simulink model "Quad_sim"  (Simulink 10.1)
settings: Solver=FixedStepAuto  StartTime=0.0  StopTime=10  FixedStep=0.01  RelTol=1e-3
values from neighbouring files (symbols this model uses):
  g = 9.81    [fcn1.m]
undefined symbols (not defined in the file or in its folder): Jr, Jx, Jy, Jz, Kd, Kd_p, Kd_q, Kd_r, Kdx, Kdy, Kdz, Ki_p, Ki_q, Ki_r, Kp_p, Kp_q, Kp_r, KT, l, m, max_motor_speed, min_motor_speed, p_max, phi_max, q_max, r_max, theta_max, U1_max, U1_min, U2_max, U2_min, U3_max, U3_min, U4_max, U4_min
settings Model: Creator=Jarvis  LastModifiedBy=nikhil
settings DataIOCC: SaveFormat=Dataset
settings OptimizationCC: LifeSpan=auto
settings DebuggingCC: UnderspecifiedInitializationDetection=Simplified  MergeDetectMultiDrivingBlocksExec=error  SFUnexpectedBacktrackingDiag=error  SFNoUnconditionalDefaultTransitionDiag=error  SFExecutionAtInitializationDiag=warning
settings HardwareCC: ProdBitPerPointer=64  ProdBitPerSizeT=64  ProdBitPerPtrDiffT=64  ProdLargestAtomicFloat=Float  ProdIntDivRoundTo=Zero  ProdEndianess=LittleEndian  ProdWordSize=64  ProdHWDeviceType=Intel->x86-64 (Windows64)
settings ModelReferenceCC: PropagateSignalLabelsOutOfModel=on
settings GRTTargetCC: TargetLangStandard=C99 (ISO)  CombineOutputUpdateFcns=on  GRTInterface=off
settings ConfigComp: CovMetricSettings=dwe  CovHtmlReporting=off  CovSaveCumulativeToWorkspaceVar=off  CovSaveSingleToWorkspaceVar=off  CovExternalEMLEnable=on

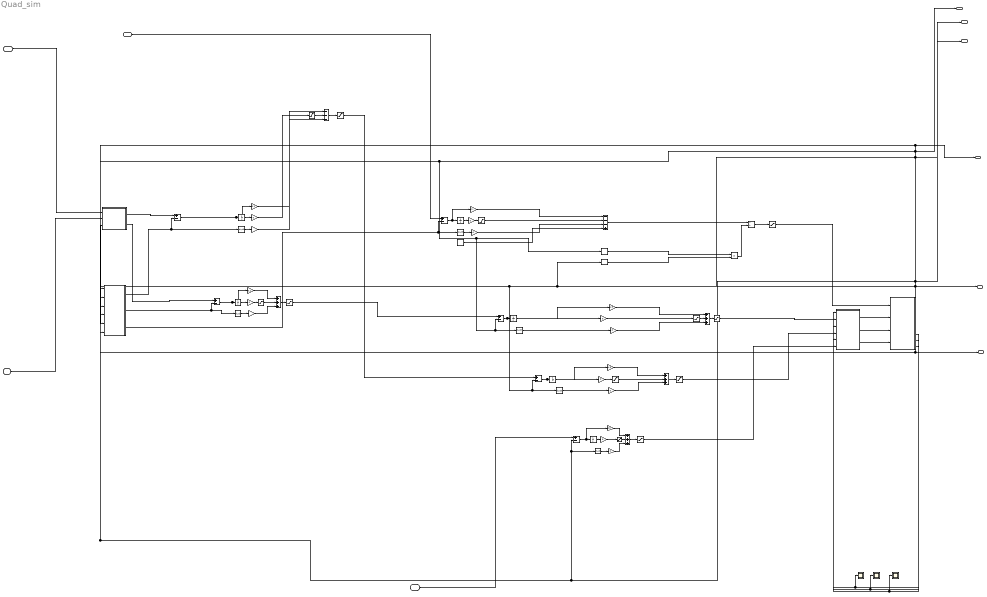
== system Quad_sim ==
  note: Psi PID
  note: Theta PID
  note: Phi PID
  note: Z PID
  note: Attitude/Altitude
      | PID Controller
  note: y control
  note: x control
  note: Position Control
  Xd : Inport
  Yd : Inport  Port=2
  Zd : Inport  Port=3
  Psid : Inport  Port=4
  Angular Rate  PID Controller : Subsystem
  "Current Positions from GF -> BF" : Subsystem
  Derivative{,1..5} (6 alike) : Derivative
  "Desired Positions from GF -> BF" : Subsystem
  Divide : Product  Inputs=*/
  Integrator{,1..5} (6 alike) : Integrator
  Kd : Gain  Gain=-0.1
  Kd1 : Gain  Gain=-0.1
  Kd2 : Gain  Gain=-4
  Kd3 : Gain  Gain=0
  Kd4 : Gain  Gain=0
  Kd5 : Gain  Gain=0
  Ki{,1..5} (6 alike) : Gain  Gain=0
  Kp : Gain  Gain=0.1
  Kp1 : Gain  Gain=0.1
  Kp2 : Gain  Gain=1.5625
  Kp3 : Gain  Gain=4.5
  Kp4 : Gain  Gain=4.5
  Kp5 : Gain  Gain=10
  Product : Product  RndMeth=Zero
  Psi Error : Sum  Inputs=+-
  Psi Error1 : Sum  Inputs=+-
  Quadrotor System : Subsystem
  Saturation : Saturate  UpperLimit=U1_max  LowerLimit=U1_min  ZeroCross=off
  Saturation1 : Saturate  UpperLimit=theta_max  LowerLimit=-theta_max  ZeroCross=off
  Saturation10 : Saturate  UpperLimit=r_max  LowerLimit=-r_max  ZeroCross=off
  Saturation11 : Saturate  UpperLimit=r_max  LowerLimit=-r_max  ZeroCross=off
  Saturation2 : Saturate  UpperLimit=theta_max  LowerLimit=-theta_max  ZeroCross=off
  Saturation3 : Saturate  UpperLimit=phi_max  LowerLimit=-phi_max  ZeroCross=off
  Saturation4 : Saturate  UpperLimit=phi_max  LowerLimit=-phi_max  ZeroCross=off
  Saturation5 : Saturate  UpperLimit=U1_max  LowerLimit=U1_min  ZeroCross=off
  Saturation6 : Saturate  UpperLimit=p_max  LowerLimit=-p_max  ZeroCross=off
  Saturation7 : Saturate  UpperLimit=p_max  LowerLimit=-p_max  ZeroCross=off
  Saturation8 : Saturate  UpperLimit=q_max  LowerLimit=-q_max  ZeroCross=off
  Saturation9 : Saturate  UpperLimit=q_max  LowerLimit=-q_max  ZeroCross=off
  Sum : Sum  Inputs=---
  Sum{1,3..5} (4 alike) : Sum  Inputs=+++
  Sum2 : Sum  Inputs=---+
  Theta Error : Sum  Inputs=+-
  X Error : Sum  Inputs=+-
  Y Error : Sum  Inputs=+-
  cos Phi : Trigonometry  Operator=cos
  cos Theta : Trigonometry  Operator=cos
  ez : Sum  Inputs=+-
  mg : Constant  Value=m*g
  p_Out : Scope
  q_Out : Scope
  r_Out : Scope
  X : Outport
  Y : Outport  Port=2
  Z : Outport  Port=3
  Phi : Outport  Port=4
  Theta : Outport  Port=5
  Psi : Outport  Port=6
  wires:
  Quadrotor System/1(Z) -> Z/1, "Current Positions from GF -> BF"/3(Z)  "Z"
  Quadrotor System/2(Phi) -> Phi/1, "Current Positions from GF -> BF"/4(phi), Psi Error/2, Derivative3/1, cos Phi/1  "Phi"
  Quadrotor System/3(Theta) -> Theta/1, "Current Positions from GF -> BF"/5(theta), Theta Error/2, Derivative4/1, cos Theta/1  "Theta"
  Quadrotor System/4(Psi) -> Psi/1, "Desired Positions from GF -> BF"/3(psi), "Current Positions from GF -> BF"/6(Psi), Psi Error1/2, Derivative5/1  "Psi"
  Quadrotor System/5(X) -> X/1, "Current Positions from GF -> BF"/1(X)  "X"
  Quadrotor System/6(Y) -> Y/1, "Current Positions from GF -> BF"/2(Y)  "Y"
  Quadrotor System/7(p) -> Angular Rate  PID Controller/1(p), p_Out/1
  Quadrotor System/8(q) -> q_Out/1, Angular Rate  PID Controller/3(q)
  Quadrotor System/9(r) -> r_Out/1, Angular Rate  PID Controller/5(r)
  Angular Rate  PID Controller/1(U2) -> Quadrotor System/2(U2)
  Angular Rate  PID Controller/2(U3) -> Quadrotor System/3(U3)
  Angular Rate  PID Controller/3(U4) -> Quadrotor System/4(U4)
  Saturation7/1 -> Angular Rate  PID Controller/2(p desired)
  Saturation9/1 -> Angular Rate  PID Controller/4(q desired)
  Saturation11/1 -> Angular Rate  PID Controller/6(r desired)
  Psid/1 -> Psi Error1/1  "Psid"
  Zd/1 -> ez/1  "Zd"
  Xd/1 -> "Desired Positions from GF -> BF"/1(X_des)  "Xd"
  Yd/1 -> "Desired Positions from GF -> BF"/2(Y_des)  "Yd"
  Saturation/1 -> Quadrotor System/1(U1)
  Sum/1 -> Saturation2/1
  Derivative/1 -> Kd/1
  Kp/1 -> Sum/1  "x_kp"
  "Desired Positions from GF -> BF"/1(x_des) -> X Error/1
  X Error/1 -> Integrator/1, Kp/1
  Saturation1/1 -> Sum/2
  Ki/1 -> Saturation1/1  "x_ki"
  "Current Positions from GF -> BF"/1(x) -> X Error/2, Derivative/1
  Kd/1 -> Sum/3  "x_kd"
  Integrator/1 -> Ki/1
  Kp1/1 -> Sum1/1  "y_kp"
  Ki1/1 -> Saturation3/1  "y_ki"
  Derivative1/1 -> Kd1/1
  "Desired Positions from GF -> BF"/2(y_des) -> Y Error/1
  Saturation3/1 -> Sum1/2
  Sum1/1 -> Saturation4/1
  "Current Positions from GF -> BF"/2(y) -> Derivative1/1, Y Error/2
  Kd1/1 -> Sum1/3  "y_kd"
  Integrator1/1 -> Ki1/1
  Y Error/1 -> Integrator1/1, Kp1/1
  Saturation5/1 -> Sum2/2
  Ki2/1 -> Saturation5/1  "z_ki"
  Divide/1 -> Saturation/1
  Kd2/1 -> Sum2/3  "z_kd"
  mg/1 -> Sum2/4
  Sum2/1 -> Divide/1
  ez/1 -> Integrator2/1, Kp2/1
  Integrator2/1 -> Ki2/1
  Kp2/1 -> Sum2/1  "z_kp"
  Derivative2/1 -> Kd2/1
  "Current Positions from GF -> BF"/3(z) -> ez/2, Derivative2/1
  Product/1 -> Divide/2
  cos Theta/1 -> Product/2
  cos Phi/1 -> Product/1
  Sum3/1 -> Saturation7/1
  Saturation6/1 -> Sum3/2
  Ki3/1 -> Saturation6/1  "phi_ki"
  Kd3/1 -> Sum3/3  "phi_kd"
  Integrator3/1 -> Ki3/1
  Psi Error/1 -> Integrator3/1, Kp3/1
  Kp3/1 -> Sum3/1  "phi_kp"
  Derivative3/1 -> Kd3/1
  Saturation4/1 -> Psi Error/1
  Sum4/1 -> Saturation9/1
  Saturation8/1 -> Sum4/2
  Ki4/1 -> Saturation8/1  "theta_ki"
  Kd4/1 -> Sum4/3  "theta_kd"
  Integrator4/1 -> Ki4/1
  Theta Error/1 -> Integrator4/1, Kp4/1
  Kp4/1 -> Sum4/1  "theta_kp"
  Derivative4/1 -> Kd4/1
  Saturation2/1 -> Theta Error/1
  Sum5/1 -> Saturation11/1
  Saturation10/1 -> Sum5/2
  Ki5/1 -> Saturation10/1  "psi_ki"
  Kd5/1 -> Sum5/3  "psi_kd"
  Integrator5/1 -> Ki5/1
  Psi Error1/1 -> Integrator5/1, Kp5/1
  Kp5/1 -> Sum5/1  "psi_kp"
  Derivative5/1 -> Kd5/1

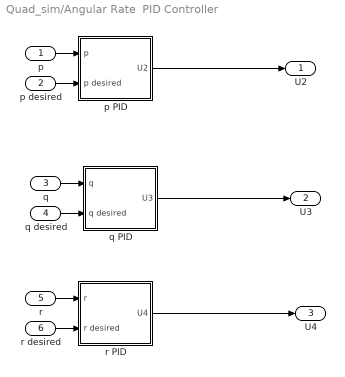
== system Quad_sim/Angular Rate  PID Controller ==
  p : Inport
  p desired : Inport  Port=2
  q : Inport  Port=3
  q desired : Inport  Port=4
  r : Inport  Port=5
  r desired : Inport  Port=6
  p PID : Subsystem
  q PID : Subsystem
  r PID : Subsystem
  U2 : Outport
  U3 : Outport  Port=2
  U4 : Outport  Port=3
  wires:
  p PID/1(U2) -> U2/1
  q PID/1(U3) -> U3/1
  r PID/1(U4) -> U4/1
  p/1 -> p PID/1(p)
  p desired/1 -> p PID/2(p desired)
  q/1 -> q PID/1(q)
  q desired/1 -> q PID/2(q desired)
  r/1 -> r PID/1(r)
  r desired/1 -> r PID/2(r desired)

== system Quad_sim/Current Positions from GF -> BF ==
  X : Inport
  Y : Inport  Port=2
  Z : Inport  Port=3
  phi : Inport  Port=4
  theta : Inport  Port=5
  Psi : Inport  Port=6
  x_bodyframe : Subsystem
  y_bodyframe : Subsystem
  z_bodyframe : Subsystem
  x : Outport
  y : Outport  Port=2
  z : Outport  Port=3
  wires:
  X/1 -> z_bodyframe/4(X), y_bodyframe/4(X), x_bodyframe/4(X)
  Y/1 -> z_bodyframe/5(Y), y_bodyframe/5(Y), x_bodyframe/5(Y)
  Z/1 -> z_bodyframe/6(Z), y_bodyframe/6(Z), x_bodyframe/6(Z)
  phi/1 -> z_bodyframe/1(phi), y_bodyframe/1(phi), x_bodyframe/1(phi)
  theta/1 -> z_bodyframe/2(theta), y_bodyframe/2(theta), x_bodyframe/2(theta)
  Psi/1 -> y_bodyframe/3(psi), x_bodyframe/3(psi), z_bodyframe/3(psi)
  x_bodyframe/1(x) -> x/1
  y_bodyframe/1(y) -> y/1
  z_bodyframe/1(z) -> z/1

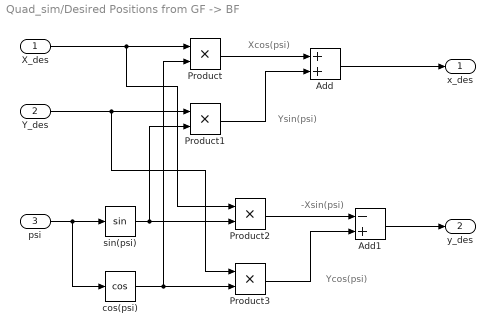
== system Quad_sim/Desired Positions from GF -> BF ==
  note: Xcos(psi)
  note: Ysin(psi)
  note: Ycos(psi)
  note: -Xsin(psi)
  X_des : Inport
  Y_des : Inport  Port=2
  psi : Inport  Port=3
  Add : Sum
  Add1 : Sum  Inputs=-+
  Product{,1..3} (4 alike) : Product
  cos(psi) : Trigonometry  Operator=cos
  sin(psi) : Trigonometry
  x_des : Outport
  y_des : Outport  Port=2
  wires:
  psi/1 -> cos(psi)/1, sin(psi)/1
  X_des/1 -> Product2/1, Product/1
  cos(psi)/1 -> Product3/2, Product/2
  Y_des/1 -> Product3/1, Product1/1
  Product/1 -> Add/1
  sin(psi)/1 -> Product2/2, Product1/2
  Product1/1 -> Add/2
  Add/1 -> x_des/1
  Product2/1 -> Add1/1
  Product3/1 -> Add1/2
  Add1/1 -> y_des/1

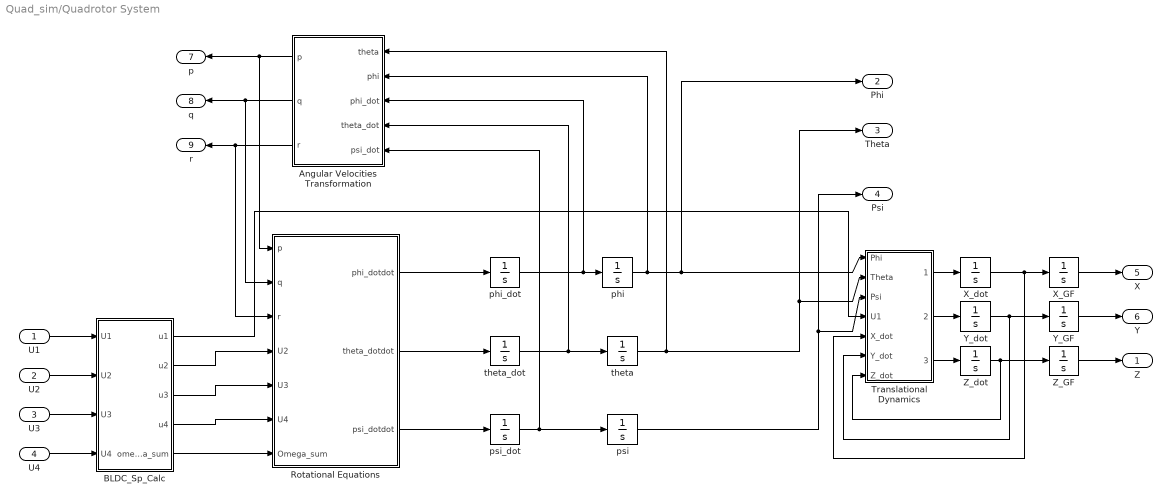
== system Quad_sim/Quadrotor System ==
  U1 : Inport
  U2 : Inport  Port=2
  U3 : Inport  Port=3
  U4 : Inport  Port=4
  Angular Velocities Transformation : Subsystem
  BLDC_Sp_Calc : Subsystem
  Rotational Equations : Subsystem
  Translational Dynamics : Subsystem
  X_GF : Integrator
  X_dot : Integrator
  Y_GF : Integrator
  Y_dot : Integrator
  Z_GF : Integrator
  Z_dot : Integrator
  phi : Integrator  ZeroCross=off
  phi_dot : Integrator
  psi : Integrator  ZeroCross=off
  psi_dot : Integrator  ZeroCross=off
  theta : Integrator  ZeroCross=off
  theta_dot : Integrator  ZeroCross=off
  Z : Outport
  Phi : Outport  Port=2
  Theta : Outport  Port=3
  Psi : Outport  Port=4
  X : Outport  Port=5
  Y : Outport  Port=6
  p : Outport  Port=7
  q : Outport  Port=8
  r : Outport  Port=9
  wires:
  U1/1 -> BLDC_Sp_Calc/1(U1)
  Angular Velocities Transformation/3(r) -> r/1, Rotational Equations/3(r)
  Angular Velocities Transformation/2(q) -> q/1, Rotational Equations/2(q)
  Angular Velocities Transformation/1(p) -> p/1, Rotational Equations/1(p)
  BLDC_Sp_Calc/4(u4) -> Rotational Equations/6(U4)
  BLDC_Sp_Calc/1(u1) -> Translational Dynamics/4(U1)
  BLDC_Sp_Calc/3(u3) -> Rotational Equations/5(U3)
  BLDC_Sp_Calc/2(u2) -> Rotational Equations/4(U2)
  U3/1 -> BLDC_Sp_Calc/3(U3)
  U2/1 -> BLDC_Sp_Calc/2(U2)
  U4/1 -> BLDC_Sp_Calc/4(U4)
  Rotational Equations/1(phi_dotdot) -> phi_dot/1
  Rotational Equations/3(psi_dotdot) -> psi_dot/1
  phi_dot/1 -> Angular Velocities Transformation/3(phi_dot), phi/1
  theta_dot/1 -> Angular Velocities Transformation/4(theta_dot), theta/1
  psi_dot/1 -> Angular Velocities Transformation/5(psi_dot), psi/1
  Z_GF/1 -> Z/1
  Y_GF/1 -> Y/1
  X_GF/1 -> X/1
  Translational Dynamics/3(z dotdot) -> Z_dot/1
  Z_dot/1 -> Z_GF/1, Translational Dynamics/7(Z_dot)
  Translational Dynamics/2(y dotdot) -> Y_dot/1
  Y_dot/1 -> Translational Dynamics/6(Y_dot), Y_GF/1
  X_dot/1 -> Translational Dynamics/5(X_dot), X_GF/1
  Translational Dynamics/1(x dotdot) -> X_dot/1
  psi/1 -> Psi/1, Translational Dynamics/3(Psi)
  theta/1 -> Angular Velocities Transformation/1(theta), Theta/1, Translational Dynamics/2(Theta)
  phi/1 -> Angular Velocities Transformation/2(phi), Phi/1, Translational Dynamics/1(Phi)
  BLDC_Sp_Calc/5(omega_sum) -> Rotational Equations/7(Omega_sum)
  Rotational Equations/2(theta_dotdot) -> theta_dot/1

== system Quad_sim/Angular Rate  PID Controller/p PID ==
  p : Inport
  p desired : Inport  Port=2
  Derivative : Derivative
  Integrator : Integrator
  Kd : Gain  Gain=Kd_p
  Ki : Gain  Gain=Ki_p
  Kp : Gain  Gain=Kp_p
  Saturation1 : Saturate  UpperLimit=U2_max  LowerLimit=U2_min  ZeroCross=off
  Saturation2 : Saturate  UpperLimit=U2_max  LowerLimit=U2_min  ZeroCross=off
  Sum : Sum  Inputs=+++
  p Error : Sum  Inputs=+-
  U2 : Outport
  wires:
  p/1 -> p Error/2, Derivative/1
  p desired/1 -> p Error/1
  Derivative/1 -> Kd/1
  Kp/1 -> Sum/1
  p Error/1 -> Integrator/1, Kp/1
  Integrator/1 -> Ki/1
  Kd/1 -> Sum/3
  Ki/1 -> Saturation1/1
  Saturation1/1 -> Sum/2
  Sum/1 -> Saturation2/1
  Saturation2/1 -> U2/1

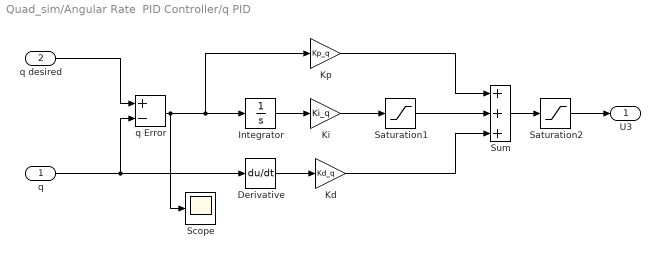
== system Quad_sim/Angular Rate  PID Controller/q PID ==
  q : Inport
  q desired : Inport  Port=2
  Derivative : Derivative
  Integrator : Integrator
  Kd : Gain  Gain=Kd_q
  Ki : Gain  Gain=Ki_q
  Kp : Gain  Gain=Kp_q
  Saturation1 : Saturate  UpperLimit=U3_max  LowerLimit=U3_min  ZeroCross=off
  Saturation2 : Saturate  UpperLimit=U3_max  LowerLimit=U3_min  ZeroCross=off
  Scope : Scope
  Sum : Sum  Inputs=+++
  q Error : Sum  Inputs=+-
  U3 : Outport
  wires:
  q/1 -> q Error/2, Derivative/1
  q desired/1 -> q Error/1
  Derivative/1 -> Kd/1
  Kp/1 -> Sum/1
  q Error/1 -> Integrator/1, Kp/1, Scope/1
  Integrator/1 -> Ki/1
  Kd/1 -> Sum/3
  Ki/1 -> Saturation1/1
  Saturation1/1 -> Sum/2
  Saturation2/1 -> U3/1
  Sum/1 -> Saturation2/1

== system Quad_sim/Angular Rate  PID Controller/r PID ==
  r : Inport
  r desired : Inport  Port=2
  Derivative : Derivative
  Integrator : Integrator
  Kd : Gain  Gain=Kd_r
  Ki : Gain  Gain=Ki_r
  Kp : Gain  Gain=Kp_r
  Saturation : Saturate  UpperLimit=U4_max  LowerLimit=U4_min  ZeroCross=off
  Saturation1 : Saturate  UpperLimit=U4_max  LowerLimit=U4_min  ZeroCross=off
  Sum : Sum  Inputs=+++
  r Error : Sum  Inputs=+-
  U4 : Outport
  wires:
  r/1 -> r Error/2, Derivative/1
  r desired/1 -> r Error/1
  Derivative/1 -> Kd/1
  Kp/1 -> Sum/1
  r Error/1 -> Integrator/1, Kp/1
  Integrator/1 -> Ki/1
  Kd/1 -> Sum/3
  Ki/1 -> Saturation/1
  Saturation/1 -> Sum/2
  Sum/1 -> Saturation1/1
  Saturation1/1 -> U4/1

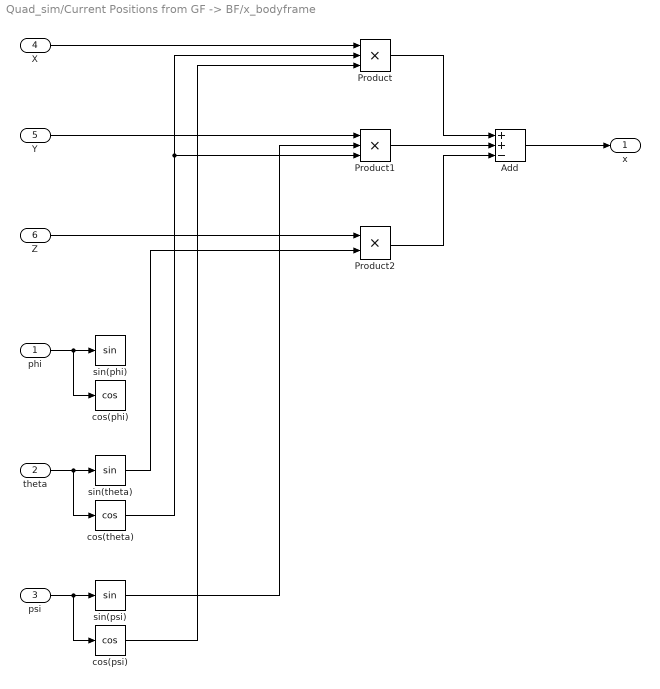
== system Quad_sim/Current Positions from GF -> BF/x_bodyframe ==
  phi : Inport
  theta : Inport  Port=2
  psi : Inport  Port=3
  X : Inport  Port=4
  Y : Inport  Port=5
  Z : Inport  Port=6
  Add : Sum  Inputs=++-
  Product : Product  Inputs=3
  Product1 : Product  Inputs=3
  Product2 : Product
  cos(phi) : Trigonometry  Operator=cos
  cos(psi) : Trigonometry  Operator=cos
  cos(theta) : Trigonometry  Operator=cos
  sin(phi) : Trigonometry
  sin(psi) : Trigonometry
  sin(theta) : Trigonometry
  x : Outport
  wires:
  theta/1 -> cos(theta)/1, sin(theta)/1
  phi/1 -> cos(phi)/1, sin(phi)/1
  psi/1 -> cos(psi)/1, sin(psi)/1
  X/1 -> Product/1
  cos(theta)/1 -> Product1/3, Product/2
  cos(psi)/1 -> Product/3
  Y/1 -> Product1/1
  sin(psi)/1 -> Product1/2
  Z/1 -> Product2/1
  sin(theta)/1 -> Product2/2
  Product1/1 -> Add/2
  Product/1 -> Add/1
  Product2/1 -> Add/3
  Add/1 -> x/1

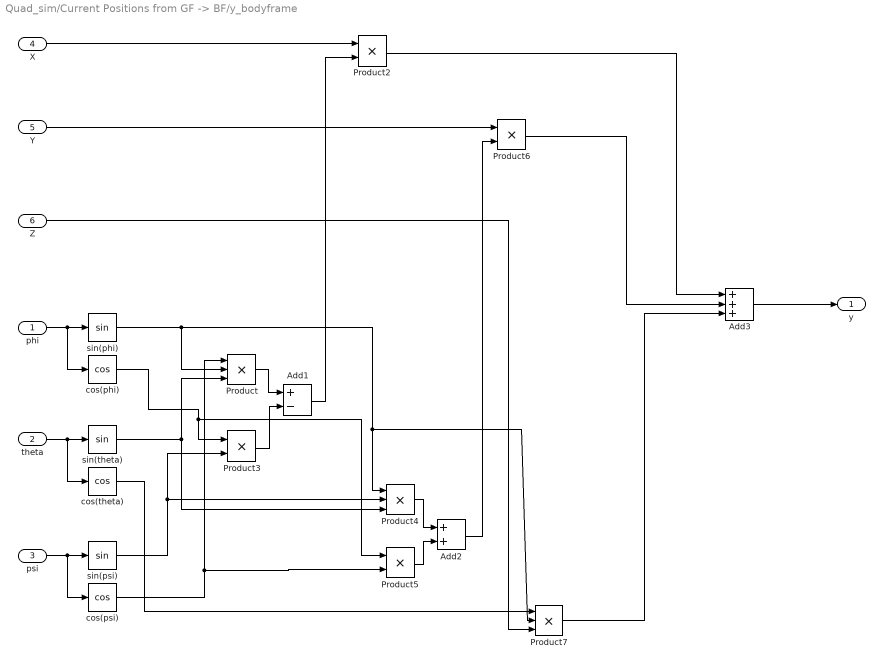
== system Quad_sim/Current Positions from GF -> BF/y_bodyframe ==
  phi : Inport
  theta : Inport  Port=2
  psi : Inport  Port=3
  X : Inport  Port=4
  Y : Inport  Port=5
  Z : Inport  Port=6
  Add1 : Sum  Inputs=+-
  Add2 : Sum
  Add3 : Sum  Inputs=+++
  Product : Product  Inputs=3
  Product{2..3,5..6} (4 alike) : Product
  Product4 : Product  Inputs=3
  Product7 : Product  Inputs=3
  cos(phi) : Trigonometry  Operator=cos
  cos(psi) : Trigonometry  Operator=cos
  cos(theta) : Trigonometry  Operator=cos
  sin(phi) : Trigonometry
  sin(psi) : Trigonometry
  sin(theta) : Trigonometry
  y : Outport
  wires:
  theta/1 -> cos(theta)/1, sin(theta)/1
  phi/1 -> cos(phi)/1, sin(phi)/1
  psi/1 -> cos(psi)/1, sin(psi)/1
  cos(psi)/1 -> Product5/2, Product/1
  sin(phi)/1 -> Product4/1, Product7/2, Product/2
  sin(theta)/1 -> Product4/3, Product/3
  cos(phi)/1 -> Product5/1, Product3/1
  sin(psi)/1 -> Product4/2, Product3/2
  Product/1 -> Add1/1
  Product3/1 -> Add1/2
  X/1 -> Product2/1
  Add1/1 -> Product2/2
  Product4/1 -> Add2/1
  Product5/1 -> Add2/2
  Add2/1 -> Product6/2
  Y/1 -> Product6/1
  cos(theta)/1 -> Product7/1
  Z/1 -> Product7/3
  Product7/1 -> Add3/3
  Product6/1 -> Add3/2
  Product2/1 -> Add3/1
  Add3/1 -> y/1

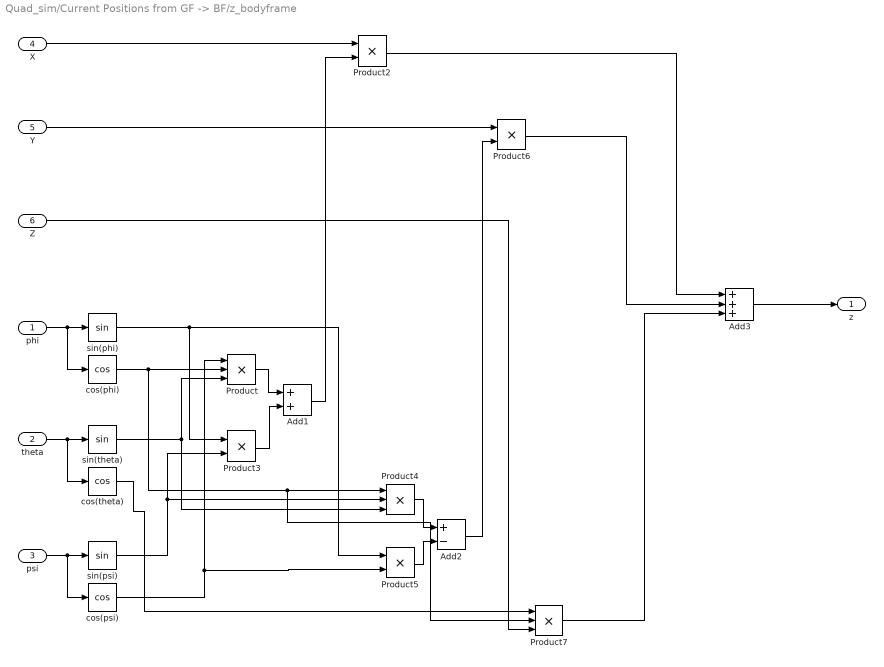
== system Quad_sim/Current Positions from GF -> BF/z_bodyframe ==
  phi : Inport
  theta : Inport  Port=2
  psi : Inport  Port=3
  X : Inport  Port=4
  Y : Inport  Port=5
  Z : Inport  Port=6
  Add1 : Sum
  Add2 : Sum  Inputs=+-
  Add3 : Sum  Inputs=+++
  Product : Product  Inputs=3
  Product{2..3,5..6} (4 alike) : Product
  Product4 : Product  Inputs=3
  Product7 : Product  Inputs=3
  cos(phi) : Trigonometry  Operator=cos
  cos(psi) : Trigonometry  Operator=cos
  cos(theta) : Trigonometry  Operator=cos
  sin(phi) : Trigonometry
  sin(psi) : Trigonometry
  sin(theta) : Trigonometry
  z : Outport
  wires:
  theta/1 -> cos(theta)/1, sin(theta)/1
  phi/1 -> cos(phi)/1, sin(phi)/1
  psi/1 -> cos(psi)/1, sin(psi)/1
  cos(psi)/1 -> Product5/2, Product/1
  sin(phi)/1 -> Product3/1, Product5/1
  sin(theta)/1 -> Product4/3, Product/3
  cos(phi)/1 -> Product/2, Product7/2, Product4/1
  sin(psi)/1 -> Product4/2, Product3/2
  Product/1 -> Add1/1
  Product3/1 -> Add1/2
  X/1 -> Product2/1
  Add1/1 -> Product2/2
  Product4/1 -> Add2/1
  Product5/1 -> Add2/2
  Add2/1 -> Product6/2
  Y/1 -> Product6/1
  cos(theta)/1 -> Product7/1
  Z/1 -> Product7/3
  Product7/1 -> Add3/3
  Product6/1 -> Add3/2
  Product2/1 -> Add3/1
  Add3/1 -> z/1

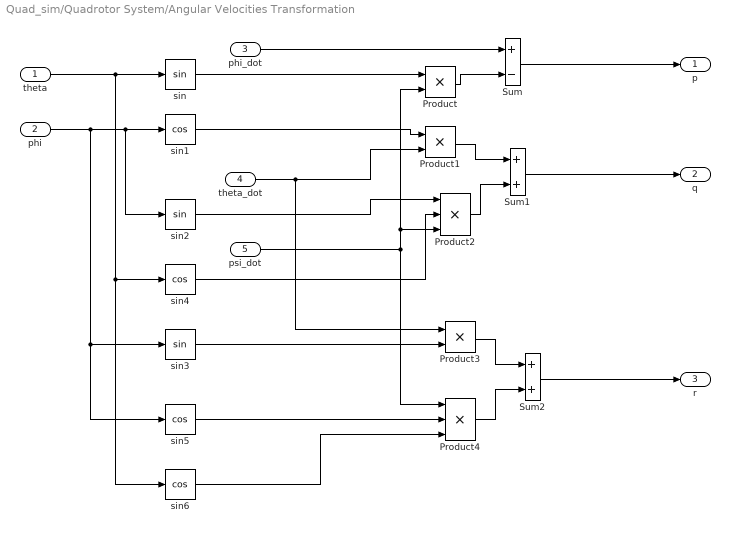
== system Quad_sim/Quadrotor System/Angular Velocities Transformation ==
  theta : Inport
  phi : Inport  Port=2
  phi_dot : Inport  Port=3
  theta_dot : Inport  Port=4
  psi_dot : Inport  Port=5
  Product : Product  RndMeth=Zero
  Product1 : Product  RndMeth=Zero
  Product2 : Product  Inputs=3  RndMeth=Zero
  Product3 : Product  RndMeth=Zero
  Product4 : Product  Inputs=3  RndMeth=Zero
  Sum : Sum  Inputs=+-
  Sum1 : Sum
  Sum2 : Sum
  sin : Trigonometry
  sin{1,4..6} (4 alike) : Trigonometry  Operator=cos
  sin2 : Trigonometry
  sin3 : Trigonometry
  p : Outport
  q : Outport  Port=2
  r : Outport  Port=3
  wires:
  Sum2/1 -> r/1
  Sum1/1 -> q/1
  Sum/1 -> p/1
  Product4/1 -> Sum2/2
  Product3/1 -> Sum2/1
  sin6/1 -> Product4/3
  sin5/1 -> Product4/2
  sin3/1 -> Product3/2
  Product2/1 -> Sum1/2
  sin4/1 -> Product2/2
  sin2/1 -> Product2/1
  Product1/1 -> Sum1/1
  theta_dot/1 -> Product3/1, Product1/2
  sin1/1 -> Product1/1
  phi/1 -> sin5/1, sin3/1, sin2/1, sin1/1
  Product/1 -> Sum/2
  psi_dot/1 -> Product4/1, Product2/3, Product/2
  sin/1 -> Product/1
  theta/1 -> sin/1, sin6/1, sin4/1
  phi_dot/1 -> Sum/1

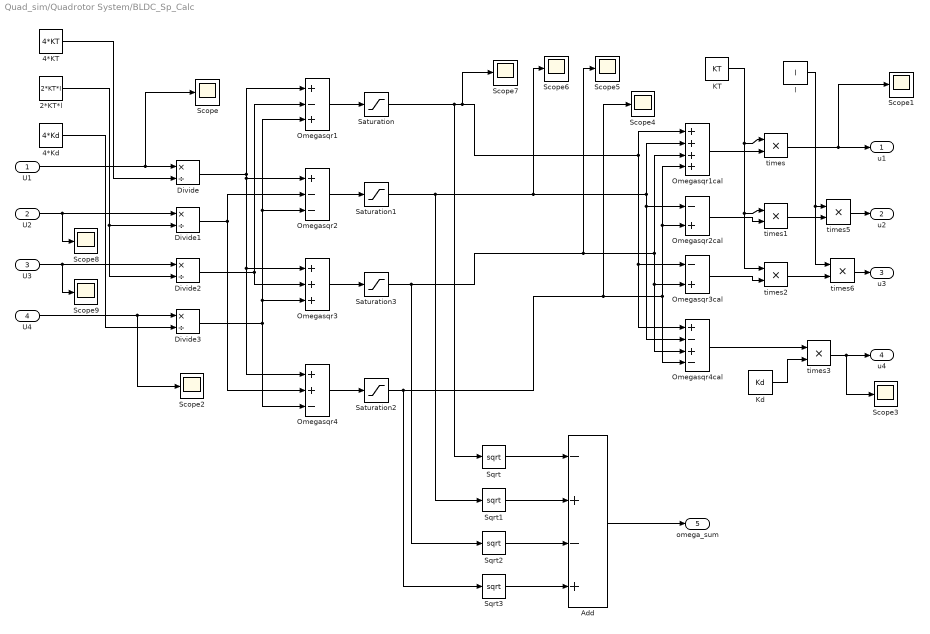
== system Quad_sim/Quadrotor System/BLDC_Sp_Calc ==
  U1 : Inport
  U2 : Inport  Port=2
  U3 : Inport  Port=3
  U4 : Inport  Port=4
  2*KT*l : Constant  Value=2*KT*l
  4*KT : Constant  Value=4*KT
  4*Kd : Constant  Value=4*Kd
  Add : Sum  Inputs=-+-+
  Divide{,1..3} (4 alike) : Product  Inputs=*/
  KT : Constant  Value=KT
  Kd : Constant  Value=Kd
  Omegasqr1 : Sum  Inputs=+-+
  Omegasqr1cal : Sum  Inputs=++++
  Omegasqr2 : Sum  Inputs=+--
  Omegasqr2cal : Sum  Inputs=-+
  Omegasqr3 : Sum  Inputs=+++
  Omegasqr3cal : Sum  Inputs=-+
  Omegasqr4 : Sum  Inputs=++-
  Omegasqr4cal : Sum  Inputs=+-+-
  Saturation{,1..3} (4 alike) : Saturate  UpperLimit=max_motor_speed^2  LowerLimit=min_motor_speed^2  ZeroCross=off
  Scope{,1..9} (10 alike) : Scope
  Sqrt{,1..3} (4 alike) : Sqrt  SaturateOnIntegerOverflow=on
  l : Constant  Value=l
  times{,1..3,5..6} (6 alike) : Product  Inputs=**
  u1 : Outport
  u2 : Outport  Port=2
  u3 : Outport  Port=3
  u4 : Outport  Port=4
  omega_sum : Outport  Port=5
  wires:
  Add/1 -> omega_sum/1
  Sqrt3/1 -> Add/4
  Sqrt2/1 -> Add/3
  Sqrt1/1 -> Add/2
  Sqrt/1 -> Add/1
  Omegasqr4/1 -> Saturation2/1
  Omegasqr3/1 -> Saturation3/1
  Omegasqr2/1 -> Saturation1/1
  Omegasqr1/1 -> Saturation/1
  Saturation1/1 -> Scope6/1, Omegasqr4cal/2, Omegasqr2cal/1, Omegasqr1cal/2, Sqrt1/1
  Saturation3/1 -> Scope5/1, Omegasqr4cal/3, Omegasqr3cal/2, Omegasqr1cal/3, Sqrt2/1
  Saturation2/1 -> Scope4/1, Omegasqr4cal/4, Omegasqr2cal/2, Omegasqr1cal/4, Sqrt3/1
  Saturation/1 -> Scope7/1, Omegasqr4cal/1, Omegasqr3cal/1, Omegasqr1cal/1, Sqrt/1
  times2/1 -> times6/2
  times1/1 -> times5/2
  l/1 -> times6/1, times5/1
  times6/1 -> u3/1
  times5/1 -> u2/1
  times3/1 -> Scope3/1, u4/1
  times/1 -> Scope1/1, u1/1
  Kd/1 -> times3/2
  Omegasqr4cal/1 -> times3/1
  Omegasqr3cal/1 -> times2/2
  Omegasqr2cal/1 -> times1/2
  Omegasqr1cal/1 -> times/2
  KT/1 -> times2/1, times1/1, times/1
  Divide1/1 -> Omegasqr4/2, Omegasqr2/2
  Divide3/1 -> Omegasqr4/3, Omegasqr3/3, Omegasqr2/3, Omegasqr1/3
  Divide2/1 -> Omegasqr3/2, Omegasqr1/2
  Divide/1 -> Omegasqr4/1, Omegasqr3/1, Omegasqr2/1, Omegasqr1/1
  4*Kd/1 -> Divide3/2
  U4/1 -> Scope2/1, Divide3/1
  U3/1 -> Scope9/1, Divide2/1
  2*KT*l/1 -> Divide2/2, Divide1/2
  U2/1 -> Scope8/1, Divide1/1
  4*KT/1 -> Divide/2
  U1/1 -> Scope/1, Divide/1

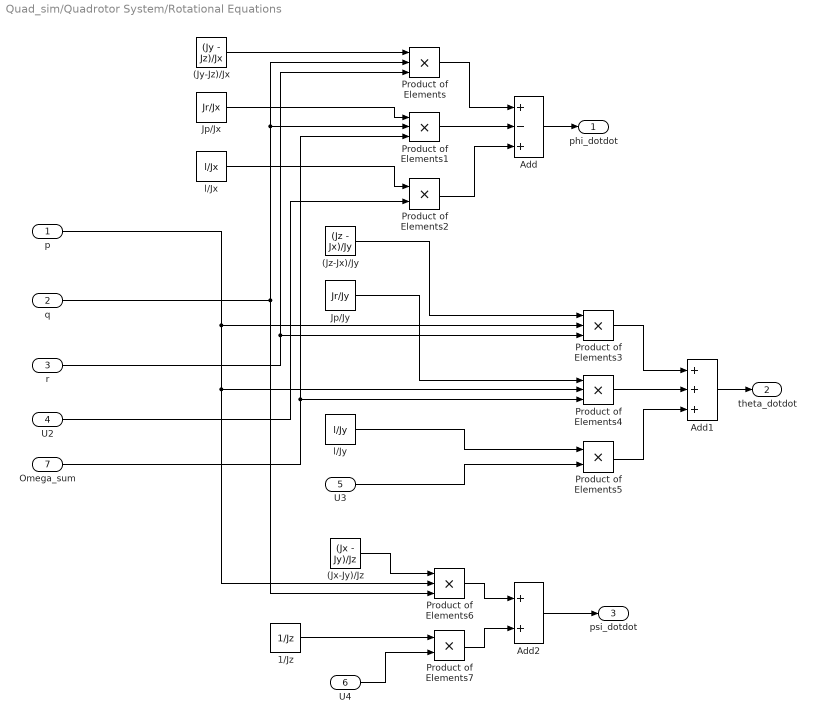
== system Quad_sim/Quadrotor System/Rotational Equations ==
  p : Inport
  q : Inport  Port=2
  r : Inport  Port=3
  U2 : Inport  Port=4
  U3 : Inport  Port=5
  U4 : Inport  Port=6
  Omega_sum : Inport  Port=7
  (Jx-Jy)/Jz : Constant  Value=(Jx - Jy)/Jz
  (Jy-Jz)/Jx : Constant  Value=(Jy - Jz)/Jx
  (Jz-Jx)/Jy : Constant  Value=(Jz - Jx)/Jy
  1/Jz : Constant  Value=1/Jz
  Add : Sum  Inputs=+-+
  Add1 : Sum  Inputs=+++
  Add2 : Sum
  Jp/Jx : Constant  Value=Jr/Jx
  Jp/Jy : Constant  Value=Jr/Jy
  Product of Elements{,1,3..4,6} (5 alike) : Product  Inputs=3
  Product of Elements2 : Product
  Product of Elements5 : Product
  Product of Elements7 : Product
  l/Jx : Constant  Value=l/Jx
  l/Jy : Constant  Value=l/Jy
  phi_dotdot : Outport
  theta_dotdot : Outport  Port=2
  psi_dotdot : Outport  Port=3
  wires:
  Product of Elements6/1 -> Add2/1
  (Jx-Jy)/Jz/1 -> Product of Elements6/1
  1/Jz/1 -> Product of Elements7/1
  U4/1 -> Product of Elements7/2
  Add2/1 -> psi_dotdot/1
  Product of Elements7/1 -> Add2/2
  p/1 -> Product of Elements6/2, Product of Elements4/2, Product of Elements3/2
  U3/1 -> Product of Elements5/2
  l/Jy/1 -> Product of Elements5/1
  Jp/Jy/1 -> Product of Elements4/1
  (Jz-Jx)/Jy/1 -> Product of Elements3/1
  Add1/1 -> theta_dotdot/1
  Product of Elements5/1 -> Add1/3
  Product of Elements4/1 -> Add1/2
  Product of Elements3/1 -> Add1/1
  Omega_sum/1 -> Product of Elements4/3, Product of Elements1/3
  U2/1 -> Product of Elements2/2
  l/Jx/1 -> Product of Elements2/1
  Jp/Jx/1 -> Product of Elements1/1
  r/1 -> Product of Elements3/3, Product of Elements/3
  q/1 -> Product of Elements6/3, Product of Elements1/2, Product of Elements/2
  (Jy-Jz)/Jx/1 -> Product of Elements/1
  Add/1 -> phi_dotdot/1
  Product of Elements2/1 -> Add/3
  Product of Elements1/1 -> Add/2
  Product of Elements/1 -> Add/1

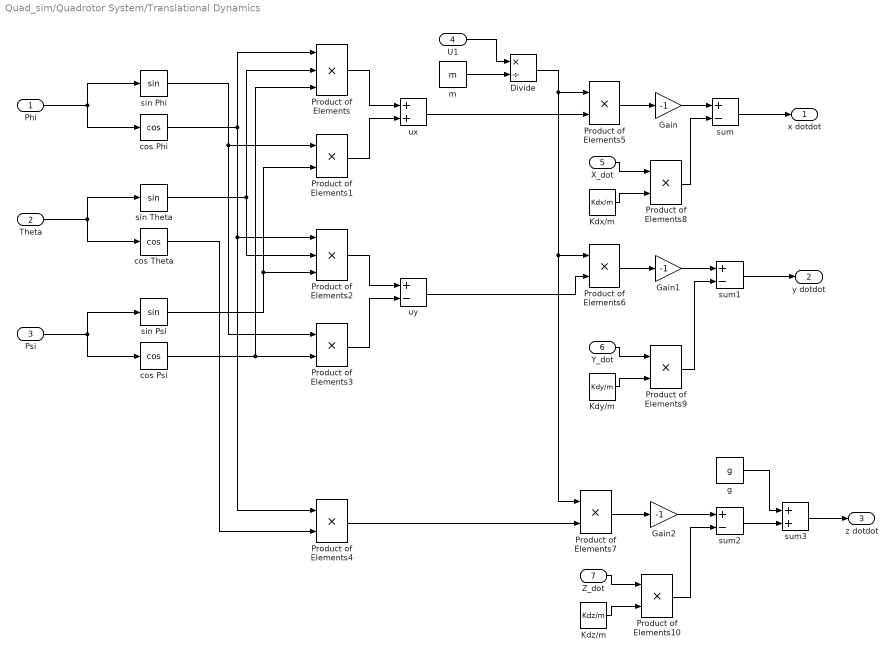
== system Quad_sim/Quadrotor System/Translational Dynamics ==
  Phi : Inport
  Theta : Inport  Port=2
  Psi : Inport  Port=3
  U1 : Inport  Port=4
  X_dot : Inport  Port=5
  Y_dot : Inport  Port=6
  Z_dot : Inport  Port=7
  Divide : Product  Inputs=*/
  Gain : Gain  Gain=-1
  Gain1 : Gain  Gain=-1
  Gain2 : Gain  Gain=-1
  Kdx/m : Constant  Value=Kdx/m
  Kdy/m : Constant  Value=Kdy/m
  Kdz/m : Constant  Value=Kdz/m
  Product of Elements : Product  Inputs=3
  Product of Elements{1,3..10} (9 alike) : Product
  Product of Elements2 : Product  Inputs=3
  cos Phi : Trigonometry  Operator=cos
  cos Psi : Trigonometry  Operator=cos
  cos Theta : Trigonometry  Operator=cos
  g : Constant  Value=g
  m : Constant  Value=m
  sin Phi : Trigonometry
  sin Psi : Trigonometry
  sin Theta : Trigonometry
  sum : Sum  Inputs=+-
  sum1 : Sum  Inputs=+-
  sum2 : Sum  Inputs=+-
  sum3 : Sum
  ux : Sum
  uy : Sum  Inputs=+-
  x dotdot : Outport
  y dotdot : Outport  Port=2
  z dotdot : Outport  Port=3
  wires:
  Gain2/1 -> sum2/1
  Product of Elements10/1 -> sum2/2
  sum2/1 -> sum3/2
  g/1 -> sum3/1
  Product of Elements7/1 -> Gain2/1
  Kdz/m/1 -> Product of Elements10/2
  Z_dot/1 -> Product of Elements10/1
  sum1/1 -> y dotdot/1
  Product of Elements9/1 -> sum1/2
  Gain1/1 -> sum1/1
  Kdy/m/1 -> Product of Elements9/2
  Y_dot/1 -> Product of Elements9/1
  sum/1 -> x dotdot/1
  Product of Elements8/1 -> sum/2
  Gain/1 -> sum/1
  Kdx/m/1 -> Product of Elements8/2
  X_dot/1 -> Product of Elements8/1
  Product of Elements6/1 -> Gain1/1
  Product of Elements5/1 -> Gain/1
  sum3/1 -> z dotdot/1
  Divide/1 -> Product of Elements7/1, Product of Elements6/1, Product of Elements5/1
  m/1 -> Divide/2
  U1/1 -> Divide/1
  Product of Elements4/1 -> Product of Elements7/2
  cos Theta/1 -> Product of Elements4/2
  uy/1 -> Product of Elements6/2
  Product of Elements3/1 -> uy/2
  Product of Elements2/1 -> uy/1
  ux/1 -> Product of Elements5/2
  Product of Elements1/1 -> ux/2
  Product of Elements/1 -> ux/1
  sin Psi/1 -> Product of Elements2/3, Product of Elements1/2
  sin Phi/1 -> Product of Elements3/1, Product of Elements1/1
  cos Phi/1 -> Product of Elements4/1, Product of Elements2/1, Product of Elements/1
  cos Psi/1 -> Product of Elements3/2, Product of Elements/3
  sin Theta/1 -> Product of Elements2/2, Product of Elements/2
  Psi/1 -> cos Psi/1, sin Psi/1
  Theta/1 -> cos Theta/1, sin Theta/1
  Phi/1 -> cos Phi/1, sin Phi/1
